simulink model "momentumBasedFlight"  (R2022b)
settings: Solver=VariableStepAuto  StartTime=0.0  StopTime=inf  RelTol=1e-3
InitFcn:
  | cd(fileparts(which(bdroot)));
  | initMomentumBasedFlight;
StopFcn:
  | cd(fileparts(which(bdroot)));
  | stopMomentumBasedFlight;
undefined symbols (not defined in the file or in its folder): aero_config, biasVectorConstraint_feet, Config, confVisualizer, ConstraintMatrix_feet, DiscIntNeverNeededParam, jets_config, robot_config
libraries: WBToolboxLibrary x20, momentum_flight_control_sublib x2, mwbs_robotDynamicsWithContacts_lib x1
(part 2 of 3)

== system momentumBasedFlight/FLIGHT CONTROLLER (CORE) V3.0/Flight Controller RAL-HUMANOIDS V3.0/Joint Torque Control for Flying/QP torqueControl ==
  HessianMatrixQP : Inport
  gVectorQP : Inport  Port=2
  ConstraintMatrix_inequality : Inport  Port=3
  biasVectorConstraint_inequality : Inport  Port=4
  feetContactIsActive : Inport  Port=5
  Constant2 : Constant  Value=Config.sat.jointTorquesSaturation
  NOT : Logic  Operator=NOT  IconShape=distinctive  AllPortsSameDT=off  OutDataTypeStr=boolean
  Process QP Inputs Torque Control : MATLAB Function  TreatAsAtomicUnit=on
  QP torqueControl - balancing : Subsystem  TreatAsAtomicUnit=on
  QP torqueControl - flight : Subsystem  TreatAsAtomicUnit=on
  Select QP torqueControl Output : Subsystem
  jointTorques_star : Outport  VectorParamsAs1DForOutWhenUnconnected=off
  exitFlagQP_torqueControl : Outport  Port=2  VectorParamsAs1DForOutWhenUnconnected=off
  wires:
  Select QP torqueControl Output/1(jointTorques_star) -> jointTorques_star/1
  Select QP torqueControl Output/2(exitFlagQP_torqueControl) -> exitFlagQP_torqueControl/1
  QP torqueControl - flight/1(QPStatus_flight) -> Select QP torqueControl Output/4(QPStatus_flight)
  QP torqueControl - flight/2(QPOutput_flight) -> Select QP torqueControl Output/5(QPOutput_flight)
  QP torqueControl - balancing/2(QPOutput_balancing) -> Select QP torqueControl Output/2(QPOutput_balancing)
  QP torqueControl - balancing/1(QPStatus_balancing) -> Select QP torqueControl Output/1(QPStatus_balancing)
  Process QP Inputs Torque Control/1(H_balancing) -> QP torqueControl - balancing/1(H)
  Process QP Inputs Torque Control/2(g_balancing) -> QP torqueControl - balancing/2(g)
  Process QP Inputs Torque Control/3(ub_balancing) -> QP torqueControl - balancing/3(ub)
  Process QP Inputs Torque Control/4(lb_balancing) -> QP torqueControl - balancing/4(lb)
  Process QP Inputs Torque Control/5(Aeq_balancing) -> QP torqueControl - balancing/5(AEq)
  Process QP Inputs Torque Control/6(lbEq_balancing) -> QP torqueControl - balancing/6(lbEq)
  Process QP Inputs Torque Control/7(ubEq_balancing) -> QP torqueControl - balancing/7(ubEq)
  Process QP Inputs Torque Control/11(lb_flight) -> QP torqueControl - flight/4(lb)
  Process QP Inputs Torque Control/10(ub_flight) -> QP torqueControl - flight/3(ub)
  Process QP Inputs Torque Control/9(g_flight) -> QP torqueControl - flight/2(g)
  Process QP Inputs Torque Control/8(H_flight) -> QP torqueControl - flight/1(H)
  Constant2/1 -> Process QP Inputs Torque Control/5(jointTorquesSaturation)
  gVectorQP/1 -> Process QP Inputs Torque Control/2(gVectorQP)
  HessianMatrixQP/1 -> Process QP Inputs Torque Control/1(HessianMatrixQP)
  ConstraintMatrix_inequality/1 -> Process QP Inputs Torque Control/3(InequalityConstrMatrix)
  biasVectorConstraint_inequality/1 -> Process QP Inputs Torque Control/4(biasVectorInequalityConstr)
  NOT/1 -> QP torqueControl - flight/Enable
  feetContactIsActive/1 -> NOT/1, QP torqueControl - balancing/Enable, Select QP torqueControl Output/3(feetContactIsActive)

== system momentumBasedFlight/FLIGHT CONTROLLER (CORE) V3.0/Flight Controller RAL-HUMANOIDS V3.0/Joint Torque Control for Flying/Torque Derivative Saturation ==
  jointTorques_star : Inport
  Constant1 : Constant  Value=Config.tStep
  Constant2 : Constant  Value=Config.sat.jointTorquesDotMax
  Saturate Torque Derivative : MATLAB Function  TreatAsAtomicUnit=on
  "holder " : WBToolboxLibrary/Utilities/holder 
      settings: SourceProductName=WholeBodyToolbox
  jointTorques_star_sat : Outport  VectorParamsAs1DForOutWhenUnconnected=off
  wires:
  Constant2/1 -> Saturate Torque Derivative/4(uDotMax)
  Constant1/1 -> Saturate Torque Derivative/3(tStep)
  "holder "/1 -> Saturate Torque Derivative/2(u_0)
  Saturate Torque Derivative/1(uSat) -> jointTorques_star_sat/1
  jointTorques_star/1 -> Saturate Torque Derivative/1(u), "holder "/1

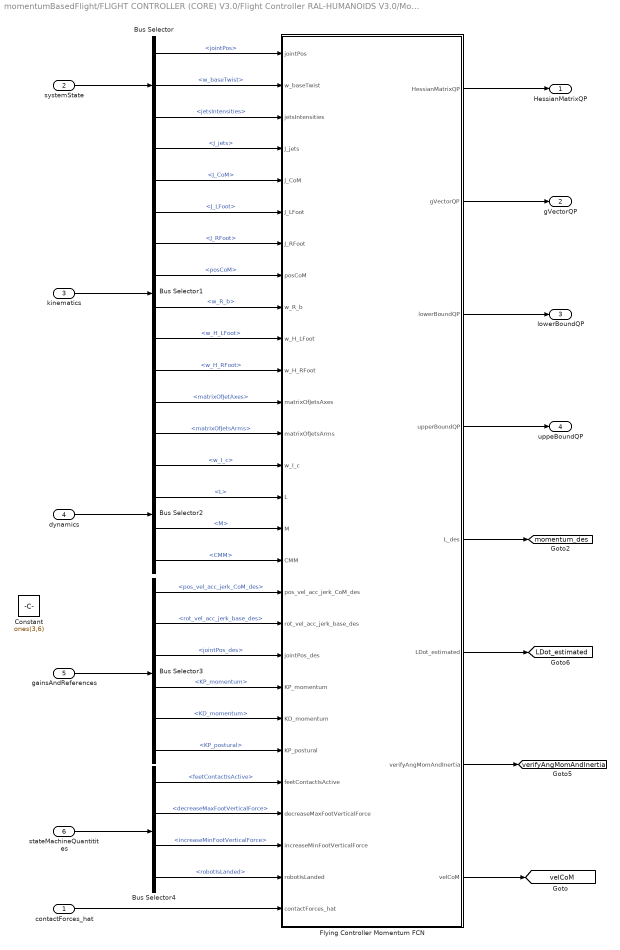
== system momentumBasedFlight/FLIGHT CONTROLLER (CORE) V3.0/Flight Controller RAL-HUMANOIDS V3.0/Momentum Control for Flying/Momentum Control ==
  contactForces_hat : Inport
  systemState : Inport  Port=2
  kinematics : Inport  Port=3
  dynamics : Inport  Port=4
  gainsAndReferences : Inport  Port=5
  stateMachineQuantitites : Inport  Port=6
  Bus Selector : BusSelector  OutputSignals=jointPos,w_baseTwist,jetsIntensities
  Bus Selector1 : BusSelector  OutputSignals=J_jets,J_CoM,J_LFoot,J_RFoot,posCoM,w_R_b,w_H_LFoot,w_H_RFoot,matrixOfJetAxes,matrixOfJetsArms
  Bus Selector2 : BusSelector  OutputSignals=w_I_c,L,M,CMM
  Bus Selector3 : BusSelector  OutputSignals=pos_vel_acc_jerk_CoM_des,rot_vel_acc_jerk_base_des,jointPos_des,KP_momentum,KD_momentum,KP_postural
  Bus Selector4 : BusSelector  OutputSignals=feetContactIsActive,decreaseMaxFootVerticalForce,increaseMinFootVerticalForce,robotIsLanded
  Constant : Constant  Value=ones(3,6)
  "Flying Controller Momentum FCN " : MATLAB Function  TreatAsAtomicUnit=on
  HessianMatrixQP : Outport  VectorParamsAs1DForOutWhenUnconnected=off
  gVectorQP : Outport  Port=2  VectorParamsAs1DForOutWhenUnconnected=off
  lowerBoundQP : Outport  Port=3  VectorParamsAs1DForOutWhenUnconnected=off
  uppeBoundQP : Outport  Port=4  VectorParamsAs1DForOutWhenUnconnected=off
  tag scope: LDot_estimated=global, momentum_des=global, velCoM=global, verifyAngMomAndInertia=global
  wires:
  "Flying Controller Momentum FCN "/8(velCoM) -> [velCoM]
  contactForces_hat/1 -> "Flying Controller Momentum FCN "/28(contactForces_hat)
  Bus Selector4/4 -> "Flying Controller Momentum FCN "/27(robotIsLanded)  "<robotIsLanded>"
  Bus Selector4/3 -> "Flying Controller Momentum FCN "/26(increaseMinFootVerticalForce)  "<increaseMinFootVerticalForce>"
  Bus Selector4/2 -> "Flying Controller Momentum FCN "/25(decreaseMaxFootVerticalForce)  "<decreaseMaxFootVerticalForce>"
  Bus Selector2/1 -> "Flying Controller Momentum FCN "/14(w_I_c)  "<w_I_c>"
  Bus Selector1/10 -> "Flying Controller Momentum FCN "/13(matrixOfJetsArms)  "<matrixOfJetsArms>"
  Bus Selector1/9 -> "Flying Controller Momentum FCN "/12(matrixOfJetsAxes)  "<matrixOfJetAxes>"
  Bus Selector3/1 -> "Flying Controller Momentum FCN "/18(pos_vel_acc_jerk_CoM_des)  "<pos_vel_acc_jerk_CoM_des>"
  Bus Selector1/6 -> "Flying Controller Momentum FCN "/9(w_R_b)  "<w_R_b>"
  Bus Selector1/5 -> "Flying Controller Momentum FCN "/8(posCoM)  "<posCoM>"
  "Flying Controller Momentum FCN "/5(L_des) -> [momentum_des]
  Bus Selector3/6 -> "Flying Controller Momentum FCN "/23(KP_postural)  "<KP_postural>"
  Bus Selector2/2 -> "Flying Controller Momentum FCN "/15(L)  "<L>"
  Bus Selector1/7 -> "Flying Controller Momentum FCN "/10(w_H_LFoot)  "<w_H_LFoot>"
  Bus Selector3/5 -> "Flying Controller Momentum FCN "/22(KD_momentum)  "<KD_momentum>"
  "Flying Controller Momentum FCN "/6(LDot_estimated) -> [LDot_estimated]
  Bus Selector2/3 -> "Flying Controller Momentum FCN "/16(M)  "<M>"
  Bus Selector2/4 -> "Flying Controller Momentum FCN "/17(CMM)  "<CMM>"
  Bus Selector1/8 -> "Flying Controller Momentum FCN "/11(w_H_RFoot)  "<w_H_RFoot>"
  Bus Selector1/4 -> "Flying Controller Momentum FCN "/7(J_RFoot)  "<J_RFoot>"
  Bus Selector/3 -> "Flying Controller Momentum FCN "/3(jetsIntensities)  "<jetsIntensities>"
  gainsAndReferences/1 -> Bus Selector3/1
  Bus Selector1/2 -> "Flying Controller Momentum FCN "/5(J_CoM)  "<J_CoM>"
  dynamics/1 -> Bus Selector2/1
  Bus Selector3/4 -> "Flying Controller Momentum FCN "/21(KP_momentum)  "<KP_momentum>"
  "Flying Controller Momentum FCN "/3(lowerBoundQP) -> lowerBoundQP/1
  stateMachineQuantitites/1 -> Bus Selector4/1
  "Flying Controller Momentum FCN "/7(verifyAngMomAndInertia) -> [verifyAngMomAndInertia]
  Bus Selector4/1 -> "Flying Controller Momentum FCN "/24(feetContactIsActive)  "<feetContactIsActive>"
  "Flying Controller Momentum FCN "/2(gVectorQP) -> gVectorQP/1
  "Flying Controller Momentum FCN "/4(upperBoundQP) -> uppeBoundQP/1
  "Flying Controller Momentum FCN "/1(HessianMatrixQP) -> HessianMatrixQP/1
  Bus Selector/2 -> "Flying Controller Momentum FCN "/2(w_baseTwist)  "<w_baseTwist>"
  Bus Selector1/1 -> "Flying Controller Momentum FCN "/4(J_jets)  "<J_jets>"
  Bus Selector/1 -> "Flying Controller Momentum FCN "/1(jointPos)  "<jointPos>"
  kinematics/1 -> Bus Selector1/1
  Bus Selector1/3 -> "Flying Controller Momentum FCN "/6(J_LFoot)  "<J_LFoot>"
  Bus Selector3/3 -> "Flying Controller Momentum FCN "/20(jointPos_des)  "<jointPos_des>"
  systemState/1 -> Bus Selector/1
  Bus Selector3/2 -> "Flying Controller Momentum FCN "/19(rot_vel_acc_jerk_base_des)  "<rot_vel_acc_jerk_base_des>"

== system momentumBasedFlight/FLIGHT CONTROLLER (CORE) V3.0/Flight Controller RAL-HUMANOIDS V3.0/Momentum Control for Flying/QP Solver and Integrate Contact Forces Derivative ==
  HessianMatrixQP : Inport
  gVectorQP : Inport  Port=2
  lowerBoundQP : Inport  Port=3
  upperBoundQP : Inport  Port=4
  stateMachineQuantities : Inport  Port=5
  systemState : Inport  Port=6
  Bus Selector1 : BusSelector  OutputSignals=feetContactIsActive
  Bus Selector2 : BusSelector  OutputSignals=contactForces
  Integrate the Contact Forces Derivative : Subsystem
  QP momentumControl : Subsystem
  contactForces_star : Outport  VectorParamsAs1DForOutWhenUnconnected=off
  jetsIntensitiesDot_star : Outport  Port=2  VectorParamsAs1DForOutWhenUnconnected=off
  jointVel_star : Outport  Port=3  VectorParamsAs1DForOutWhenUnconnected=off
  tag scope: contactForces_star=global, exitFlagQP_momentumControl=global, jetsIntensitiesDot_star=global, jointVel_star=global
  wires:
  systemState/1 -> Bus Selector2/1
  Bus Selector2/1 -> Integrate the Contact Forces Derivative/2(contactForces)  "<contactForces>"
  Bus Selector1/1 -> Integrate the Contact Forces Derivative/3(feetContactIsActive), QP momentumControl/5(feetContactIsActive)  "<feetContactIsActive>"
  QP momentumControl/3(jointVel_star) -> jointVel_star/1, [jointVel_star]
  QP momentumControl/1(jetsIntensitiesDot_star) -> jetsIntensitiesDot_star/1, [jetsIntensitiesDot_star]
  HessianMatrixQP/1 -> QP momentumControl/1(HessianMatrixQP)
  stateMachineQuantities/1 -> Bus Selector1/1
  gVectorQP/1 -> QP momentumControl/2(gVectorQP)
  QP momentumControl/4(exitFlagQP_momentumControl) -> [exitFlagQP_momentumControl]
  upperBoundQP/1 -> QP momentumControl/4(upperBoundQP)
  lowerBoundQP/1 -> QP momentumControl/3(lowerBoundQP)
  Integrate the Contact Forces Derivative/1(contactForces_star) -> contactForces_star/1, [contactForces_star]
  QP momentumControl/2(contactForcesDot_star) -> Integrate the Contact Forces Derivative/1(contactForcesDot_star)

== system momentumBasedFlight/FLIGHT CONTROLLER (CORE) V3.0/Jets Control/extendedKalmanFilter4jets/EKF_jet1 ==
  input : Inport
  jetIntensityMeasurement : Inport  Port=2
  Constant : Constant  Value=[Config.initT, Config.initTdot]
  Constant1 : Constant  Value=Config.ekf.initP
  Discrete-Time Integrator1 : DiscreteIntegrator  InitialConditionSource=external  SampleTime=Config.tStep  ICPrevOutput=DiscIntNeverNeededParam  ICPrevScaledInput=DiscIntNeverNeededParam
  Discrete-Time Integrator2 : DiscreteIntegrator  InitialConditionSource=external  SampleTime=Config.tStep  ICPrevOutput=DiscIntNeverNeededParam  ICPrevScaledInput=DiscIntNeverNeededParam
  "EKF " : MATLAB Function  TreatAsAtomicUnit=on
  splitVector : MATLAB Function  TreatAsAtomicUnit=on
  jetIntensityFiltered : Outport  VectorParamsAs1DForOutWhenUnconnected=off
  jetDerivativeEstimated : Outport  Port=2  VectorParamsAs1DForOutWhenUnconnected=off
  wires:
  splitVector/2(x2) -> jetDerivativeEstimated/1
  splitVector/1(x1) -> jetIntensityFiltered/1
  Constant1/1 -> Discrete-Time Integrator2/2
  Discrete-Time Integrator2/1 -> "EKF "/4(P)
  jetIntensityMeasurement/1 -> "EKF "/3(measurement)
  Constant/1 -> Discrete-Time Integrator1/2
  Discrete-Time Integrator1/1 -> splitVector/1(x), "EKF "/1(x)
  input/1 -> "EKF "/2(input)
  "EKF "/1(xDot) -> Discrete-Time Integrator1/1
  "EKF "/2(Pdot) -> Discrete-Time Integrator2/1

== system momentumBasedFlight/FLIGHT CONTROLLER (CORE) V3.0/Jets Control/extendedKalmanFilter4jets/EKF_jet2 ==
  input : Inport
  jetIntensityMeasurement : Inport  Port=2
  Constant : Constant  Value=[Config.initT, Config.initTdot]
  Constant1 : Constant  Value=Config.ekf.initP
  Discrete-Time Integrator1 : DiscreteIntegrator  InitialConditionSource=external  SampleTime=Config.tStep  ICPrevOutput=DiscIntNeverNeededParam  ICPrevScaledInput=DiscIntNeverNeededParam
  Discrete-Time Integrator2 : DiscreteIntegrator  InitialConditionSource=external  SampleTime=Config.tStep  ICPrevOutput=DiscIntNeverNeededParam  ICPrevScaledInput=DiscIntNeverNeededParam
  "EKF " : MATLAB Function  TreatAsAtomicUnit=on
  splitVector : MATLAB Function  TreatAsAtomicUnit=on
  jetIntensityFiltered : Outport  VectorParamsAs1DForOutWhenUnconnected=off
  jetDerivativeEstimated : Outport  Port=2  VectorParamsAs1DForOutWhenUnconnected=off
  wires:
  "EKF "/2(Pdot) -> Discrete-Time Integrator2/1
  "EKF "/1(xDot) -> Discrete-Time Integrator1/1
  input/1 -> "EKF "/2(input)
  Discrete-Time Integrator1/1 -> "EKF "/1(x), splitVector/1(x)
  Constant/1 -> Discrete-Time Integrator1/2
  jetIntensityMeasurement/1 -> "EKF "/3(measurement)
  Discrete-Time Integrator2/1 -> "EKF "/4(P)
  Constant1/1 -> Discrete-Time Integrator2/2
  splitVector/1(x1) -> jetIntensityFiltered/1
  splitVector/2(x2) -> jetDerivativeEstimated/1

== system momentumBasedFlight/FLIGHT CONTROLLER (CORE) V3.0/Jets Control/extendedKalmanFilter4jets/EKF_jet3 ==
  input : Inport
  jetIntensityMeasurement : Inport  Port=2
  Constant : Constant  Value=[Config.initT, Config.initTdot]
  Constant1 : Constant  Value=Config.ekf.initP
  Discrete-Time Integrator1 : DiscreteIntegrator  InitialConditionSource=external  SampleTime=Config.tStep  ICPrevOutput=DiscIntNeverNeededParam  ICPrevScaledInput=DiscIntNeverNeededParam
  Discrete-Time Integrator2 : DiscreteIntegrator  InitialConditionSource=external  SampleTime=Config.tStep  ICPrevOutput=DiscIntNeverNeededParam  ICPrevScaledInput=DiscIntNeverNeededParam
  "EKF " : MATLAB Function  TreatAsAtomicUnit=on
  splitVector : MATLAB Function  TreatAsAtomicUnit=on
  jetIntensityFiltered : Outport  VectorParamsAs1DForOutWhenUnconnected=off
  jetDerivativeEstimated : Outport  Port=2  VectorParamsAs1DForOutWhenUnconnected=off
  wires:
  splitVector/2(x2) -> jetDerivativeEstimated/1
  splitVector/1(x1) -> jetIntensityFiltered/1
  Constant1/1 -> Discrete-Time Integrator2/2
  Discrete-Time Integrator2/1 -> "EKF "/4(P)
  jetIntensityMeasurement/1 -> "EKF "/3(measurement)
  Constant/1 -> Discrete-Time Integrator1/2
  Discrete-Time Integrator1/1 -> splitVector/1(x), "EKF "/1(x)
  input/1 -> "EKF "/2(input)
  "EKF "/1(xDot) -> Discrete-Time Integrator1/1
  "EKF "/2(Pdot) -> Discrete-Time Integrator2/1

== system momentumBasedFlight/FLIGHT CONTROLLER (CORE) V3.0/Jets Control/extendedKalmanFilter4jets/EKF_jet4 ==
  input : Inport
  jetIntensityMeasurement : Inport  Port=2
  Constant : Constant  Value=[Config.initT, Config.initTdot]
  Constant1 : Constant  Value=Config.ekf.initP
  Discrete-Time Integrator1 : DiscreteIntegrator  InitialConditionSource=external  SampleTime=Config.tStep  ICPrevOutput=DiscIntNeverNeededParam  ICPrevScaledInput=DiscIntNeverNeededParam
  Discrete-Time Integrator2 : DiscreteIntegrator  InitialConditionSource=external  SampleTime=Config.tStep  ICPrevOutput=DiscIntNeverNeededParam  ICPrevScaledInput=DiscIntNeverNeededParam
  "EKF " : MATLAB Function  TreatAsAtomicUnit=on
  splitVector : MATLAB Function  TreatAsAtomicUnit=on
  jetIntensityFiltered : Outport  VectorParamsAs1DForOutWhenUnconnected=off
  jetDerivativeEstimated : Outport  Port=2  VectorParamsAs1DForOutWhenUnconnected=off
  wires:
  "EKF "/2(Pdot) -> Discrete-Time Integrator2/1
  "EKF "/1(xDot) -> Discrete-Time Integrator1/1
  input/1 -> "EKF "/2(input)
  Discrete-Time Integrator1/1 -> "EKF "/1(x), splitVector/1(x)
  Constant/1 -> Discrete-Time Integrator1/2
  jetIntensityMeasurement/1 -> "EKF "/3(measurement)
  Discrete-Time Integrator2/1 -> "EKF "/4(P)
  Constant1/1 -> Discrete-Time Integrator2/2
  splitVector/1(x1) -> jetIntensityFiltered/1
  splitVector/2(x2) -> jetDerivativeEstimated/1

== system momentumBasedFlight/iRonCub/Forward Dynamics/jetsDyn/Simulink Function ==
  simFunc_getFrameFreeFloatingJacobianJet1Frame : TriggerPort  TriggerType=function-call  IsSimulinkFunction=on  FunctionName=simFunc_getFrameFreeFloatingJacobianJet1Frame  FunctionVisibility=scoped  VariantControl=(inherit)
  Jacobian Left Foot : WBToolboxLibrary/Model/Jacobians/Jacobian  frameName=Frames.JET1_FRAME
      settings: SourceProductName=WholeBodyToolbox
  basePose : ArgIn  DisableCoverage=on  PortDimensions=[4,4]  ArgumentName=basePose
  jointPosition : ArgIn  Port=2  PortDimensions=[robot_config.N_DOF,1]  ArgumentName=jointPosition
  jacobian : ArgOut  DisableCoverage=on  PortDimensions=[6,6+robot_config.N_DOF]  ArgumentName=jacobian
  wires:
  Jacobian Left Foot/1 -> jacobian/1
  jointPosition/1 -> Jacobian Left Foot/2
  basePose/1 -> Jacobian Left Foot/1

== system momentumBasedFlight/iRonCub/Forward Dynamics/jetsDyn/Simulink Function1 ==
  simFunc_getWorldTransformJet2Frame : TriggerPort  TriggerType=function-call  IsSimulinkFunction=on  FunctionName=simFunc_getWorldTransformJet2Frame  FunctionVisibility=scoped  VariantControl=(inherit)
  ForwardKinematics : WBToolboxLibrary/Model/Kinematics/ForwardKinematics  frameName=Frames.JET2_FRAME
      settings: SourceProductName=WholeBodyToolbox
  basePose : ArgIn  DisableCoverage=on  PortDimensions=[4,4]  ArgumentName=basePose
  jointPosition : ArgIn  Port=2  PortDimensions=[robot_config.N_DOF,1]  ArgumentName=jointPosition
  w_H_jet2Frame : ArgOut  DisableCoverage=on  PortDimensions=[4,4]  ArgumentName=w_H_jet2Frame
  wires:
  ForwardKinematics/1 -> w_H_jet2Frame/1
  jointPosition/1 -> ForwardKinematics/2
  basePose/1 -> ForwardKinematics/1

== system momentumBasedFlight/iRonCub/Forward Dynamics/jetsDyn/Simulink Function2 ==
  simFunc_getWorldTransformJet3Frame : TriggerPort  TriggerType=function-call  IsSimulinkFunction=on  FunctionName=simFunc_getWorldTransformJet3Frame  FunctionVisibility=scoped  VariantControl=(inherit)
  ForwardKinematics : WBToolboxLibrary/Model/Kinematics/ForwardKinematics  frameName=Frames.JET3_FRAME
      settings: SourceProductName=WholeBodyToolbox
  basePose : ArgIn  DisableCoverage=on  PortDimensions=[4,4]  ArgumentName=basePose
  jointPosition : ArgIn  Port=2  PortDimensions=[robot_config.N_DOF,1]  ArgumentName=jointPosition
  w_H_jet3Frame : ArgOut  DisableCoverage=on  PortDimensions=[4,4]  ArgumentName=w_H_jet3Frame
  wires:
  ForwardKinematics/1 -> w_H_jet3Frame/1
  jointPosition/1 -> ForwardKinematics/2
  basePose/1 -> ForwardKinematics/1

== system momentumBasedFlight/iRonCub/Forward Dynamics/jetsDyn/Simulink Function3 ==
  simFunc_getWorldTransformJet4Frame : TriggerPort  TriggerType=function-call  IsSimulinkFunction=on  FunctionName=simFunc_getWorldTransformJet4Frame  FunctionVisibility=scoped  VariantControl=(inherit)
  ForwardKinematics : WBToolboxLibrary/Model/Kinematics/ForwardKinematics  frameName=Frames.JET4_FRAME
      settings: SourceProductName=WholeBodyToolbox
  basePose : ArgIn  DisableCoverage=on  PortDimensions=[4,4]  ArgumentName=basePose
  jointPosition : ArgIn  Port=2  PortDimensions=[robot_config.N_DOF,1]  ArgumentName=jointPosition
  w_H_jet4Frame : ArgOut  DisableCoverage=on  PortDimensions=[4,4]  ArgumentName=w_H_jet4Frame
  wires:
  basePose/1 -> ForwardKinematics/1
  jointPosition/1 -> ForwardKinematics/2
  ForwardKinematics/1 -> w_H_jet4Frame/1

== system momentumBasedFlight/iRonCub/Forward Dynamics/jetsDyn/Simulink Function4 ==
  simFunc_getFrameFreeFloatingJacobianJet2Frame : TriggerPort  TriggerType=function-call  IsSimulinkFunction=on  FunctionName=simFunc_getFrameFreeFloatingJacobianJet2Frame  FunctionVisibility=scoped  VariantControl=(inherit)
  Jacobian Left Foot : WBToolboxLibrary/Model/Jacobians/Jacobian  frameName=Frames.JET2_FRAME
      settings: SourceProductName=WholeBodyToolbox
  basePose : ArgIn  DisableCoverage=on  PortDimensions=[4,4]  ArgumentName=basePose
  jointPosition : ArgIn  Port=2  PortDimensions=[robot_config.N_DOF,1]  ArgumentName=jointPosition
  jacobian : ArgOut  DisableCoverage=on  PortDimensions=[6,6+robot_config.N_DOF]  ArgumentName=jacobian
  wires:
  Jacobian Left Foot/1 -> jacobian/1
  jointPosition/1 -> Jacobian Left Foot/2
  basePose/1 -> Jacobian Left Foot/1

== system momentumBasedFlight/iRonCub/Forward Dynamics/jetsDyn/Simulink Function5 ==
  simFunc_getFrameFreeFloatingJacobianJet3Frame : TriggerPort  TriggerType=function-call  IsSimulinkFunction=on  FunctionName=simFunc_getFrameFreeFloatingJacobianJet3Frame  FunctionVisibility=scoped  VariantControl=(inherit)
  Jacobian Left Foot : WBToolboxLibrary/Model/Jacobians/Jacobian  frameName=Frames.JET3_FRAME
      settings: SourceProductName=WholeBodyToolbox
  basePose : ArgIn  DisableCoverage=on  PortDimensions=[4,4]  ArgumentName=basePose
  jointPosition : ArgIn  Port=2  PortDimensions=[robot_config.N_DOF,1]  ArgumentName=jointPosition
  jacobian : ArgOut  DisableCoverage=on  PortDimensions=[6,6+robot_config.N_DOF]  ArgumentName=jacobian
  wires:
  Jacobian Left Foot/1 -> jacobian/1
  jointPosition/1 -> Jacobian Left Foot/2
  basePose/1 -> Jacobian Left Foot/1

== system momentumBasedFlight/iRonCub/Forward Dynamics/jetsDyn/Simulink Function6 ==
  simFunc_getFrameFreeFloatingJacobianJet4Frame : TriggerPort  TriggerType=function-call  IsSimulinkFunction=on  FunctionName=simFunc_getFrameFreeFloatingJacobianJet4Frame  FunctionVisibility=scoped  VariantControl=(inherit)
  Jacobian Left Foot : WBToolboxLibrary/Model/Jacobians/Jacobian  frameName=Frames.JET4_FRAME
      settings: SourceProductName=WholeBodyToolbox
  basePose : ArgIn  DisableCoverage=on  PortDimensions=[4,4]  ArgumentName=basePose
  jointPosition : ArgIn  Port=2  PortDimensions=[robot_config.N_DOF,1]  ArgumentName=jointPosition
  jacobian : ArgOut  DisableCoverage=on  PortDimensions=[6,6+robot_config.N_DOF]  ArgumentName=jacobian
  wires:
  Jacobian Left Foot/1 -> jacobian/1
  jointPosition/1 -> Jacobian Left Foot/2
  basePose/1 -> Jacobian Left Foot/1

== system momentumBasedFlight/iRonCub/Forward Dynamics/jetsDyn/Simulink Function7 ==
  simFunc_getWorldTransformJet1Frame : TriggerPort  TriggerType=function-call  IsSimulinkFunction=on  FunctionName=simFunc_getWorldTransformJet1Frame  FunctionVisibility=scoped  VariantControl=(inherit)
  ForwardKinematics : WBToolboxLibrary/Model/Kinematics/ForwardKinematics  frameName=Frames.JET1_FRAME
      settings: SourceProductName=WholeBodyToolbox
  basePose : ArgIn  DisableCoverage=on  PortDimensions=[4,4]  ArgumentName=basePose
  jointPosition : ArgIn  Port=2  PortDimensions=[robot_config.N_DOF,1]  ArgumentName=jointPosition
  w_H_jet1Frame : ArgOut  DisableCoverage=on  PortDimensions=[4,4]  ArgumentName=w_H_jet1Frame
  wires:
  basePose/1 -> ForwardKinematics/1
  jointPosition/1 -> ForwardKinematics/2
  ForwardKinematics/1 -> w_H_jet1Frame/1

== system momentumBasedFlight/FLIGHT CONTROLLER (CORE) V3.0/Flight Controller RAL-HUMANOIDS V3.0/Joint Torque Control for Flying/QP torqueControl/QP torqueControl - balancing ==
  H : Inport
  g : Inport  Port=2
  ub : Inport  Port=3
  lb : Inport  Port=4
  AEq : Inport  Port=5
  lbEq : Inport  Port=6
  ubEq : Inport  Port=7
  Enable : EnablePort
  Combine Bounds and Inequalities : MATLAB Function  TreatAsAtomicUnit=on
  MatchSignalSizes : WBToolboxLibrary/Utilities/MatchSignalSizes
      settings: SourceProductName=WholeBodyToolbox
  QP balancing-torqueControl : WBToolboxLibrary/Utilities/QP  lbA=on  ubA=on  lb=off  ub=off  computeObjVal=off  stopIfFails=off
      settings: SourceProductName=WholeBodyToolbox
  QPStatus_balancing : Outport  VectorParamsAs1DForOutWhenUnconnected=off
  QPOutput_balancing : Outport  Port=2  VectorParamsAs1DForOutWhenUnconnected=off
  wires:
  Combine Bounds and Inequalities/3(ubEq_combined) -> QP balancing-torqueControl/5
  Combine Bounds and Inequalities/2(lbEq_combined) -> QP balancing-torqueControl/4
  Combine Bounds and Inequalities/1(AEq_combined) -> QP balancing-torqueControl/3
  ub/1 -> Combine Bounds and Inequalities/5(ub)
  lb/1 -> Combine Bounds and Inequalities/4(lb)
  ubEq/1 -> Combine Bounds and Inequalities/3(ubEq)
  lbEq/1 -> Combine Bounds and Inequalities/2(lbEq)
  AEq/1 -> Combine Bounds and Inequalities/1(AEq)
  g/1 -> QP balancing-torqueControl/2, MatchSignalSizes/1
  H/1 -> QP balancing-torqueControl/1
  QP balancing-torqueControl/1 -> MatchSignalSizes/2
  MatchSignalSizes/1 -> QPOutput_balancing/1
  QP balancing-torqueControl/2 -> QPStatus_balancing/1

== system momentumBasedFlight/FLIGHT CONTROLLER (CORE) V3.0/Flight Controller RAL-HUMANOIDS V3.0/Joint Torque Control for Flying/QP torqueControl/QP torqueControl - flight ==
  H : Inport
  g : Inport  Port=2
  ub : Inport  Port=3
  lb : Inport  Port=4
  Enable : EnablePort
  Constant : Constant  Value=eye(Config.N_DOF)
  MatchSignalSizes : WBToolboxLibrary/Utilities/MatchSignalSizes
      settings: SourceProductName=WholeBodyToolbox
  QP flight-torqueControl : WBToolboxLibrary/Utilities/QP  lbA=on  ubA=on  lb=off  ub=off  computeObjVal=off  stopIfFails=off
      settings: SourceProductName=WholeBodyToolbox
  QPStatus_flight : Outport  VectorParamsAs1DForOutWhenUnconnected=off
  QPOutput_flight : Outport  Port=2  VectorParamsAs1DForOutWhenUnconnected=off
  wires:
  ub/1 -> QP flight-torqueControl/5
  g/1 -> MatchSignalSizes/1, QP flight-torqueControl/2
  H/1 -> QP flight-torqueControl/1
  QP flight-torqueControl/1 -> MatchSignalSizes/2
  MatchSignalSizes/1 -> QPOutput_flight/1
  lb/1 -> QP flight-torqueControl/4
  QP flight-torqueControl/2 -> QPStatus_flight/1
  Constant/1 -> QP flight-torqueControl/3

== system momentumBasedFlight/FLIGHT CONTROLLER (CORE) V3.0/Flight Controller RAL-HUMANOIDS V3.0/Joint Torque Control for Flying/QP torqueControl/Select QP torqueControl Output ==
  QPStatus_balancing : Inport
  QPOutput_balancing : Inport  Port=2
  feetContactIsActive : Inport  Port=3
  QPStatus_flight : Inport  Port=4
  QPOutput_flight : Inport  Port=5
  Demux : Demux  Outputs=[12;Config.N_DOF]
  Switch : Switch  Criteria=u2 > Threshold  SaturateOnIntegerOverflow=off  InputSameDT=off
  Switch1 : Switch  Criteria=u2 > Threshold  SaturateOnIntegerOverflow=off  InputSameDT=off
  contactForces_QP : Terminator
  jointTorques_star : Outport  VectorParamsAs1DForOutWhenUnconnected=off
  exitFlagQP_torqueControl : Outport  Port=2  VectorParamsAs1DForOutWhenUnconnected=off
  wires:
  Demux/2 -> Switch1/1
  Demux/1 -> contactForces_QP/1
  QPOutput_flight/1 -> Switch1/3
  QPOutput_balancing/1 -> Demux/1
  Switch/1 -> exitFlagQP_torqueControl/1
  QPStatus_flight/1 -> Switch/3
  QPStatus_balancing/1 -> Switch/1
  feetContactIsActive/1 -> Switch/2, Switch1/2
  Switch1/1 -> jointTorques_star/1

== system momentumBasedFlight/FLIGHT CONTROLLER (CORE) V3.0/Flight Controller RAL-HUMANOIDS V3.0/Momentum Control for Flying/QP Solver and Integrate Contact Forces Derivative/Integrate the Contact Forces Derivative ==
  contactForcesDot_star : Inport
  contactForces : Inport  Port=2
  feetContactIsActive : Inport  Port=3
  Discrete-Time Integrator1 : DiscreteIntegrator  ExternalReset=either  InitialConditionSource=external  InitialCondition=zeros(6,1)  SampleTime=Config.tStep  ICPrevOutput=DiscIntNeverNeededParam  ICPrevScaledInput=DiscIntNeverNeededParam
  Select Integrator Initial Condition : MATLAB Function  TreatAsAtomicUnit=on
  deadZone : Subsystem
  contactForces_star : Outport  VectorParamsAs1DForOutWhenUnconnected=off
  tag scope: contactForcesDot_star=global
  wires:
  Select Integrator Initial Condition/1(contactForces_0) -> Discrete-Time Integrator1/3
  feetContactIsActive/1 -> Discrete-Time Integrator1/2, Select Integrator Initial Condition/1(feetContactIsActive)
  contactForces/1 -> Select Integrator Initial Condition/2(contactForces)
  deadZone/1(u_cut) -> Discrete-Time Integrator1/1
  contactForcesDot_star/1 -> [contactForcesDot_star], deadZone/1(u)
  Discrete-Time Integrator1/1 -> contactForces_star/1

== system momentumBasedFlight/FLIGHT CONTROLLER (CORE) V3.0/Flight Controller RAL-HUMANOIDS V3.0/Momentum Control for Flying/QP Solver and Integrate Contact Forces Derivative/QP momentumControl ==
  HessianMatrixQP : Inport
  gVectorQP : Inport  Port=2
  lowerBoundQP : Inport  Port=3
  upperBoundQP : Inport  Port=4
  feetContactIsActive : Inport  Port=5
  NOT : Logic  Operator=NOT  IconShape=distinctive  AllPortsSameDT=off  OutDataTypeStr=boolean
  Process QP Inputs Momentum Control : MATLAB Function  TreatAsAtomicUnit=on
  QP momentumControl - balancing : Subsystem  TreatAsAtomicUnit=on
  QP momentumControl - flight : Subsystem  TreatAsAtomicUnit=on
  Select QP momentumControl Output : Subsystem
  jetsIntensitiesDot_star : Outport  VectorParamsAs1DForOutWhenUnconnected=off
  contactForcesDot_star : Outport  Port=2  VectorParamsAs1DForOutWhenUnconnected=off
  jointVel_star : Outport  Port=3  VectorParamsAs1DForOutWhenUnconnected=off
  exitFlagQP_momentumControl : Outport  Port=4  VectorParamsAs1DForOutWhenUnconnected=off
  wires:
  QP momentumControl - flight/2(QPOutput_flight) -> Select QP momentumControl Output/5(QPOutput_flight)
  QP momentumControl - flight/1(QPStatus_flight) -> Select QP momentumControl Output/4(QPStatus_flight)
  QP momentumControl - balancing/2(QPOutput_balancing) -> Select QP momentumControl Output/2(QPOutput_balancing)
  QP momentumControl - balancing/1(QPStatus_balancing) -> Select QP momentumControl Output/1(QPStatus_balancing)
  Select QP momentumControl Output/4(exitFlagQP_momentumControl) -> exitFlagQP_momentumControl/1
  NOT/1 -> QP momentumControl - flight/Enable
  Process QP Inputs Momentum Control/8(lb_flight) -> QP momentumControl - flight/4(lb)
  Process QP Inputs Momentum Control/7(ub_flight) -> QP momentumControl - flight/3(ub)
  Process QP Inputs Momentum Control/4(lb_balancing) -> QP momentumControl - balancing/4(lb)
  Process QP Inputs Momentum Control/3(ub_balancing) -> QP momentumControl - balancing/3(ub)
  Process QP Inputs Momentum Control/6(g_flight) -> QP momentumControl - flight/2(g)
  Process QP Inputs Momentum Control/5(H_flight) -> QP momentumControl - flight/1(H)
  Process QP Inputs Momentum Control/2(g_balancing) -> QP momentumControl - balancing/2(g)
  Process QP Inputs Momentum Control/1(H_balancing) -> QP momentumControl - balancing/1(H)
  Select QP momentumControl Output/2(contactForcesDot_star) -> contactForcesDot_star/1
  Select QP momentumControl Output/3(jointVel_star) -> jointVel_star/1
  Select QP momentumControl Output/1(jetsIntensitiesDot_star) -> jetsIntensitiesDot_star/1
  HessianMatrixQP/1 -> Process QP Inputs Momentum Control/1(HessianMatrixQP)
  upperBoundQP/1 -> Process QP Inputs Momentum Control/4(upperBoundQP)
  feetContactIsActive/1 -> QP momentumControl - balancing/Enable, NOT/1, Select QP momentumControl Output/3(feetContactIsActive)
  lowerBoundQP/1 -> Process QP Inputs Momentum Control/3(lowerBoundQP)
  gVectorQP/1 -> Process QP Inputs Momentum Control/2(gVectorQP)

== system momentumBasedFlight/FLIGHT CONTROLLER (CORE) V3.0/Flight Controller RAL-HUMANOIDS V3.0/Momentum Control for Flying/QP Solver and Integrate Contact Forces Derivative/Integrate the Contact Forces Derivative/deadZone ==
  u : Inport
  Constant : Constant  Value=Config.sat.deadZoneThreshold
  Deadzone Function : MATLAB Function  TreatAsAtomicUnit=on
  u_cut : Outport  VectorParamsAs1DForOutWhenUnconnected=off
  wires:
  Constant/1 -> Deadzone Function/2(thr)
  u/1 -> Deadzone Function/1(u)
  Deadzone Function/1(y) -> u_cut/1

== system momentumBasedFlight/FLIGHT CONTROLLER (CORE) V3.0/Flight Controller RAL-HUMANOIDS V3.0/Momentum Control for Flying/QP Solver and Integrate Contact Forces Derivative/QP momentumControl/QP momentumControl - balancing ==
  H : Inport
  g : Inport  Port=2
  ub : Inport  Port=3
  lb : Inport  Port=4
  Enable : EnablePort
  Constant : Constant  Value=eye(Config.N_DOF + 12 + 4)
  MatchSignalSizes : WBToolboxLibrary/Utilities/MatchSignalSizes
      settings: SourceProductName=WholeBodyToolbox
  QP : WBToolboxLibrary/Utilities/QP  lbA=on  ubA=on  lb=off  ub=off  computeObjVal=off  stopIfFails=off
      settings: SourceProductName=WholeBodyToolbox
  QPStatus_balancing : Outport  VectorParamsAs1DForOutWhenUnconnected=off
  QPOutput_balancing : Outport  Port=2  VectorParamsAs1DForOutWhenUnconnected=off
  wires:
  ub/1 -> QP/5
  QP/1 -> MatchSignalSizes/2
  MatchSignalSizes/1 -> QPOutput_balancing/1
  QP/2 -> QPStatus_balancing/1
  H/1 -> QP/1
  g/1 -> MatchSignalSizes/1, QP/2
  lb/1 -> QP/4
  Constant/1 -> QP/3

== system momentumBasedFlight/FLIGHT CONTROLLER (CORE) V3.0/Flight Controller RAL-HUMANOIDS V3.0/Momentum Control for Flying/QP Solver and Integrate Contact Forces Derivative/QP momentumControl/QP momentumControl - flight ==
  H : Inport
  g : Inport  Port=2
  ub : Inport  Port=3
  lb : Inport  Port=4
  Enable : EnablePort
  Constant : Constant  Value=eye(Config.N_DOF + 4)
  MatchSignalSizes : WBToolboxLibrary/Utilities/MatchSignalSizes
      settings: SourceProductName=WholeBodyToolbox
  QP flight-momentumControl : WBToolboxLibrary/Utilities/QP  lbA=on  ubA=on  lb=off  ub=off  computeObjVal=off  stopIfFails=off
      settings: SourceProductName=WholeBodyToolbox
  QPStatus_flight : Outport  VectorParamsAs1DForOutWhenUnconnected=off
  QPOutput_flight : Outport  Port=2  VectorParamsAs1DForOutWhenUnconnected=off
  wires:
  ub/1 -> QP flight-momentumControl/5
  g/1 -> MatchSignalSizes/1, QP flight-momentumControl/2
  H/1 -> QP flight-momentumControl/1
  QP flight-momentumControl/1 -> MatchSignalSizes/2
  MatchSignalSizes/1 -> QPOutput_flight/1
  lb/1 -> QP flight-momentumControl/4
  QP flight-momentumControl/2 -> QPStatus_flight/1
  Constant/1 -> QP flight-momentumControl/3

== system momentumBasedFlight/FLIGHT CONTROLLER (CORE) V3.0/Flight Controller RAL-HUMANOIDS V3.0/Momentum Control for Flying/QP Solver and Integrate Contact Forces Derivative/QP momentumControl/Select QP momentumControl Output ==
  QPStatus_balancing : Inport
  QPOutput_balancing : Inport  Port=2
  feetContactIsActive : Inport  Port=3
  QPStatus_flight : Inport  Port=4
  QPOutput_flight : Inport  Port=5
  Constant : Constant  Value=zeros(12,1)
  Demux : Demux  Outputs=[4;12;Config.N_DOF]
  Demux1 : Demux  Outputs=[4;Config.N_DOF]
  Switch{,1..3} (4 alike) : Switch  Criteria=u2 > Threshold  SaturateOnIntegerOverflow=off  InputSameDT=off
  jetsIntensitiesDot_star : Outport  VectorParamsAs1DForOutWhenUnconnected=off
  contactForcesDot_star : Outport  Port=2  VectorParamsAs1DForOutWhenUnconnected=off
  jointVel_star : Outport  Port=3  VectorParamsAs1DForOutWhenUnconnected=off
  exitFlagQP_momentumControl : Outport  Port=4  VectorParamsAs1DForOutWhenUnconnected=off
  wires:
  Demux1/2 -> Switch3/3
  Demux/3 -> Switch3/1
  Constant/1 -> Switch2/3
  Demux/2 -> Switch2/1
  Demux1/1 -> Switch1/3
  Demux/1 -> Switch1/1
  QPOutput_flight/1 -> Demux1/1
  QPOutput_balancing/1 -> Demux/1
  Switch/1 -> exitFlagQP_momentumControl/1
  QPStatus_flight/1 -> Switch/3
  QPStatus_balancing/1 -> Switch/1
  feetContactIsActive/1 -> Switch/2, Switch1/2, Switch2/2, Switch3/2
  Switch3/1 -> jointVel_star/1
  Switch1/1 -> jetsIntensitiesDot_star/1
  Switch2/1 -> contactForcesDot_star/1

== matlab function momentumBasedFlight/FLIGHT CONTROLLER (CORE) V3.0/Flight Controller RAL-HUMANOIDS V3.0/Joint Torque Control for Flying/QP torqueControl/Process QP Inputs Torque Control ==
  data: HessianMatrixQP input; H_balancing output; gVectorQP input; InequalityConstrMatrix input; biasVectorInequalityConstr input; g_balancing output; ub_balancing output; lb_balancing output; Aeq_balancing output; lbEq_balancing output; ubEq_balancing output; H_flight output; g_flight output; ub_flight output; lb_flight output; jointTorquesSaturation input; Config parameter
function [H_balancing,g_balancing,ub_balancing,lb_balancing,Aeq_balancing,lbEq_balancing,ubEq_balancing, ...
          H_flight,g_flight,ub_flight,lb_flight] = processQPinputTorqueControlFCN ...
                                                       (HessianMatrixQP,gVectorQP,InequalityConstrMatrix, ...
                                                        biasVectorInequalityConstr,jointTorquesSaturation,Config)   
   
[H_balancing,g_balancing,ub_balancing,lb_balancing,Aeq_balancing,lbEq_balancing,ubEq_balancing, ...
          H_flight,g_flight,ub_flight,lb_flight] = iRonCubLib.processQPinputTorqueControl ...
                                                       (HessianMatrixQP,gVectorQP,InequalityConstrMatrix, ...
                                                        biasVectorInequalityConstr,jointTorquesSaturation,Config);     
end

== matlab function momentumBasedFlight/FLIGHT CONTROLLER (CORE) V3.0/Flight Controller RAL-HUMANOIDS V3.0/Joint Torque Control for Flying/QP torqueControl/QP torqueControl - balancing/Combine Bounds and Inequalities ==
  data: AEq input; AEq_combined output; lbEq input; ubEq input; lb input; ub input; lbEq_combined output; ubEq_combined output
function [AEq_combined,lbEq_combined,ubEq_combined] = combineInputBoundsAndInequalitiesQPFCN(AEq,lbEq,ubEq,lb,ub)

   [AEq_combined,lbEq_combined,ubEq_combined] = iRonCubLib.combineInputBoundsAndInequalitiesQP(AEq,lbEq,ubEq,lb,ub);
end

== matlab function momentumBasedFlight/FLIGHT CONTROLLER (CORE) V3.0/Jets Control/extendedKalmanFilter4jets/EKF_jet1/EKF  ==
  data: x input; input input; measurement input; xDot output; P input; Config parameter; Pdot output
function [xDot, Pdot] = extendedKalmanFilterFNC(x, input, measurement, P, Config)

[xDot, Pdot] = extKalmanFilter(x, input, Config.jetC_P100, P, measurement, Config);

== matlab function momentumBasedFlight/FLIGHT CONTROLLER (CORE) V3.0/Flight Controller RAL-HUMANOIDS V3.0/Joint Torque Control for Flying/torqueControlFCN ==
  data: M input; h input; J_jets input; J_LFoot input; J_RFoot input; JDot_LFoot_nu input; JDot_RFoot_nu input; w_H_LFoot input; w_H_RFoot input; matrixOfJetsAxes input; ConstraintsMatrix_feet input; biasVectorConstraint_feet input; jetsIntensities input; stateVel input; jointVel_star input; contactForces_star input; KI_torqueControl input; KP_torqueControl input; feetContactIsActive input; activateEqConstrTorqueControl input; robotIsLanded input; jointPos_err input; Hessian output; Config parameter; gradient output; ConstraintMatrix_inequality output; biasVectorConstraint_inequality output; jointVel_err output
function [Hessian, gradient, ConstraintMatrix_inequality, biasVectorConstraint_inequality, jointVel_err] =  ... 
             flyingTorqueControlFCN(M, h, J_jets, J_LFoot, J_RFoot, JDot_LFoot_nu, JDot_RFoot_nu, w_H_LFoot, w_H_RFoot, matrixOfJetsAxes, ...
                                    ConstraintsMatrix_feet, biasVectorConstraint_feet, jetsIntensities, stateVel, jointVel_star, contactForces_star, ...
                                    KI_torqueControl, KP_torqueControl, feetContactIsActive, activateEqConstrTorqueControl, robotIsLanded, jointPos_err, Config)
                                      
    [Hessian, gradient, ConstraintMatrix_inequality, biasVectorConstraint_inequality, jointVel_err] =  ... 
        iRonCubLib.flyingTorqueControl(M, h, J_jets, J_LFoot, J_RFoot, JDot_LFoot_nu, JDot_RFoot_nu, w_H_LFoot, w_H_RFoot, matrixOfJetsAxes, ...
                                       ConstraintsMatrix_feet, biasVectorConstraint_feet, jetsIntensities, stateVel, jointVel_star, contactForces_star, ...
                                       KI_torqueControl, KP_torqueControl, feetContactIsActive, activateEqConstrTorqueControl, robotIsLanded, jointPos_err, Config);           
end

== matlab function momentumBasedFlight/FLIGHT CONTROLLER (CORE) V3.0/Flight Controller RAL-HUMANOIDS V3.0/Momentum Control for Flying/Momentum Control/Flying Controller Momentum FCN  ==
  data: jointPos input; w_baseTwist input; jetsIntensities input; J_jets input; J_CoM input; J_LFoot input; J_RFoot input; posCoM input; w_R_b input; w_H_LFoot input; w_H_RFoot input; matrixOfJetsAxes input; matrixOfJetsArms input; w_I_c input; L input; M input; CMM input; pos_vel_acc_jerk_CoM_des input; rot_vel_acc_jerk_base_des input size=[3,6]; jointPos_des input; KP_momentum input; KD_momentum input; KP_postural input; feetContactIsActive input; decreaseMaxFootVerticalForce input; increaseMinFootVerticalForce input; robotIsLanded input; HessianMatrixQP output; gVectorQP output; lowerBoundQP output; upperBoundQP output; L_des output; LDot_estimated output; verifyAngMomAndInertia output; contactForces_hat input; Config parameter; velCoM output
function [HessianMatrixQP, gVectorQP, lowerBoundQP, upperBoundQP, L_des, LDot_estimated, verifyAngMomAndInertia, velCoM] = ...
             flyingMomentumControlFCN(jointPos, w_baseTwist, jetsIntensities, J_jets, J_CoM, J_LFoot, J_RFoot, posCoM, w_R_b, w_H_LFoot, ...
                                      w_H_RFoot, matrixOfJetsAxes, matrixOfJetsArms, w_I_c, L, M, CMM, pos_vel_acc_jerk_CoM_des, ....
                                      rot_vel_acc_jerk_base_des, jointPos_des, KP_momentum, KD_momentum, KP_postural, feetContactIsActive, ...
                                      decreaseMaxFootVerticalForce, increaseMinFootVerticalForce, robotIsLanded, contactForces_hat, Config)
                               
    [HessianMatrixQP, gVectorQP, lowerBoundQP, upperBoundQP, L_des, LDot_estimated, verifyAngMomAndInertia, velCoM] = ...
        iRonCubLib.flyingMomentumControl(jointPos, w_baseTwist, jetsIntensities, J_jets, J_CoM, J_LFoot, J_RFoot, posCoM, w_R_b, w_H_LFoot, ...
                                         w_H_RFoot, matrixOfJetsAxes, matrixOfJetsArms, w_I_c, L, M, CMM, pos_vel_acc_jerk_CoM_des, ...
                                         rot_vel_acc_jerk_base_des, jointPos_des, KP_momentum, KD_momentum, KP_postural, feetContactIsActive, ...
                                         decreaseMaxFootVerticalForce, increaseMinFootVerticalForce, robotIsLanded, contactForces_hat, Config);
end

== matlab function momentumBasedFlight/FLIGHT CONTROLLER (CORE) V3.0/Jets Control/extendedKalmanFilter4jets/EKF_jet1/splitVector ==
  data: x input; x1 output; x2 output
function [x1, x2] = fcn(x)
x1 = x(1);
x2 = x(2);

== matlab function momentumBasedFlight/Visualizer1/Task and Base Frame Kinematics/Get RPY error norm ==
  data: rot_err input; rotErr_norm output
function rotErr_norm = normFCN(rot_err)

rotErr_norm = norm(rot_err);

end

== matlab function momentumBasedFlight/FLIGHT CONTROLLER (CORE) V3.0/Flight Controller RAL-HUMANOIDS V3.0/Momentum Control for Flying/QP Solver and Integrate Contact Forces Derivative/Integrate the Contact Forces Derivative/Select Integrator Initial Condition ==
  data: feetContactIsActive input; contactForces input; contactForces_0 output
function contactForces_0 = selectInitContactForcesFCN(feetContactIsActive, contactForces)

    contactForces_0 = iRonCubLib.selectInitContactForces(feetContactIsActive, contactForces);
end

== matlab function momentumBasedFlight/FLIGHT CONTROLLER (CORE) V3.0/Jets Control/extendedKalmanFilter4jets/EKF_jet2/EKF  ==
  data: x input; input input; measurement input; xDot output; P input; Config parameter; Pdot output
function [xDot, Pdot] = extendedKalmanFilterFNC(x, input, measurement, P, Config)

[xDot, Pdot] = extKalmanFilter(x, input, Config.jetC_P100, P, measurement, Config);

== matlab function momentumBasedFlight/FLIGHT CONTROLLER (CORE) V3.0/JoyStick-flightGUI Commands/Replace Joystick with Native GUI ==
  data: gui_input input; joyButtons output; joyAxes output
function [joyButtons,joyAxes] = fromGuiToJoystickFCN(gui_input)

    [joyButtons,joyAxes] = iRonCubLib.fromGuiToJoystick(gui_input);
end

== matlab function momentumBasedFlight/FLIGHT CONTROLLER (CORE) V3.0/Get System State/Change Contact Forces Representation/Change Contact Forces Representation ==
  data: contactForces_WBD input; mixed_f_l_sole output; w_R_l_sole input; w_R_r_sole input; mixed_f_r_sole output
function [mixed_f_l_sole, mixed_f_r_sole] = fromBodyFrameToMixed_contactForcesFCN(contactForces_WBD, w_R_l_sole, w_R_r_sole)

    [mixed_f_l_sole, mixed_f_r_sole] = iRonCubLib.fromBodyFrameToMixed_contactForces(contactForces_WBD, w_R_l_sole, w_R_r_sole);
end

== matlab function momentumBasedFlight/Visualizer1/Task and Base Frame Kinematics/Get RPY from rotation matrix ==
  data: w_R_b input; rollPitchYaw output
function rollPitchYaw = rollPitchYawFromRotationFCN(w_R_b)

rollPitchYaw = wbc.rollPitchYawFromRotation(w_R_b);

end

== matlab function momentumBasedFlight/Visualizer1/Task and Base Frame Kinematics/Get RPY from rotation matrix  ==
  data: w_R_b input; rollPitchYaw output
function rollPitchYaw = rollPitchYawFromRotationFCN(w_R_b)

rollPitchYaw = wbc.rollPitchYawFromRotation(w_R_b);

end

== matlab function momentumBasedFlight/Visualizer1/Task and Base Frame Kinematics/MATLAB Function1 ==
  data: RPY_Corr output; rollPitchYaw input
function RPY_Corr = correctYawAngleFCN(rollPitchYaw)

    RPY_Corr = correctYawAngle(rollPitchYaw);

end

== matlab function momentumBasedFlight/FLIGHT CONTROLLER (CORE) V3.0/Jets Control/extendedKalmanFilter4jets/EKF_jet2/splitVector ==
  data: x input; x1 output; x2 output
function [x1, x2] = fcn(x)
x1 = x(1);
x2 = x(2);

== matlab function momentumBasedFlight/FLIGHT CONTROLLER (CORE) V3.0/Jets Control/extendedKalmanFilter4jets/EKF_jet3/EKF  ==
  data: x input; input input; measurement input; xDot output; P input; Config parameter; Pdot output
function [xDot, Pdot] = extendedKalmanFilterFNC(x, input, measurement, P, Config)

[xDot, Pdot] = extKalmanFilter(x, input, Config.jetC_P220, P, measurement, Config);

== matlab function momentumBasedFlight/Visualizer1/Task and Base Frame Kinematics/MATLAB Function2 ==
  data: RPY_Corr output; rollPitchYaw input
function RPY_Corr = correctYawAngleFCN(rollPitchYaw)

    RPY_Corr = correctYawAngle(rollPitchYaw);

end

== matlab function momentumBasedFlight/FLIGHT CONTROLLER (CORE) V3.0/Jets Control/extendedKalmanFilter4jets/EKF_jet3/splitVector ==
  data: x input; x1 output; x2 output
function [x1, x2] = fcn(x)
x1 = x(1);
x2 = x(2);

== matlab function momentumBasedFlight/Visualizer1/Task and Base Frame Kinematics/MATLAB Function3 ==
  data: RPY_Corr output; rollPitchYaw input
function RPY_Corr = correctYawAngleFCN(rollPitchYaw)

    RPY_Corr = correctYawAngle(rollPitchYaw);

end

== matlab function momentumBasedFlight/iRonCub/Forward Dynamics/jetsDyn/MATLAB Function ==
  data: u input; u1 output; u2 output; u3 output; u4 output
function [u1, u2, u3, u4] = splitVec(u)
u1 = u(1);
u2 = u(2);
u3 = u(3);
u4 = u(4);

== matlab function momentumBasedFlight/FLIGHT CONTROLLER (CORE) V3.0/Jets Control/extendedKalmanFilter4jets/EKF_jet4/EKF  ==
  data: x input; input input; measurement input; xDot output; P input; Config parameter; Pdot output
function [xDot, Pdot] = extendedKalmanFilterFNC(x, input, measurement, P, Config)

[xDot, Pdot] = extKalmanFilter(x, input, Config.jetC_P220, P, measurement, Config);

== matlab function momentumBasedFlight/FLIGHT CONTROLLER (CORE) V3.0/Jets Control/extendedKalmanFilter4jets/EKF_jet4/splitVector ==
  data: x input; x1 output; x2 output
function [x1, x2] = fcn(x)
x1 = x(1);
x2 = x(2);

== matlab function momentumBasedFlight/FLIGHT CONTROLLER (CORE) V3.0/Flight Controller RAL-HUMANOIDS V3.0/Momentum Control for Flying/QP Solver and Integrate Contact Forces Derivative/Integrate the Contact Forces Derivative/deadZone/Deadzone Function ==
  data: u input; y output; thr input
function y = deadZoneFCN(u, thr)

    y = wbc.deadZone(u, thr);
end

== matlab function momentumBasedFlight/FLIGHT CONTROLLER (CORE) V3.0/Flight Controller RAL-HUMANOIDS V3.0/Momentum Control for Flying/QP Solver and Integrate Contact Forces Derivative/QP momentumControl/Process QP Inputs Momentum Control ==
  data: HessianMatrixQP input; H_balancing output; gVectorQP input; lowerBoundQP input; upperBoundQP input; g_balancing output; ub_balancing output; lb_balancing output; H_flight output; g_flight output; ub_flight output; lb_flight output
function [H_balancing,g_balancing,ub_balancing,lb_balancing, ...
          H_flight,g_flight,ub_flight,lb_flight] = processQPinputMomentumControlFCN(HessianMatrixQP,gVectorQP,lowerBoundQP,upperBoundQP) 
      
    [H_balancing,g_balancing,ub_balancing,lb_balancing, ...
        H_flight,g_flight,ub_flight,lb_flight] = iRonCubLib.processQPinputMomentumControl(HessianMatrixQP,gVectorQP,lowerBoundQP,upperBoundQP);
end

== matlab function momentumBasedFlight/FLIGHT CONTROLLER (CORE) V3.0/Flight Controller RAL-HUMANOIDS V3.0/Joint Torque Control for Flying/Torque Derivative Saturation/Saturate Torque Derivative ==
  data: u input; uSat output; u_0 input; tStep input; uDotMax input
function uSat = saturateInputDerivativeFCN(u, u_0, tStep, uDotMax)

    uSat = wbc.saturateInputDerivative(u, u_0, tStep, uDotMax);
end
